simulink subsystem "Dynamics_6DOF_QUAT"  (R2024b)
settings: Solver=VariableStepAuto  StartTime=0.0  StopTime=10.0  RelTol=1e-3
undefined symbols (not defined in the file): Earth, F, fractalcoef, GC, GlobalPosition, Light, MIL, Parameters, WGS84
libraries: aerolibwind2 x3, sharedtransform x2, robotcorelib x2, shared6dof x1, aerolibatmos2 x1, mspfiltlib x1, simulink x1, aerolibasang x1, aerolibtransform2 x1, eeGeneralControl x1, simulink_extras x1, sensorgpslib x1
settings Model: Creator=thesa  LastModifiedBy=jack
settings RTWCC: GPUComputeCapability=3.5

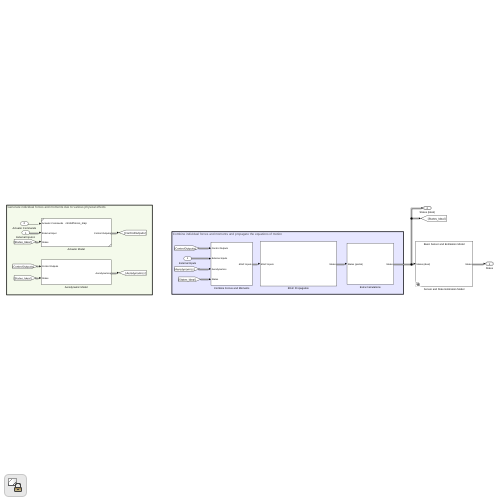
[thumbnail: Simulink's stored preview of the top-level diagram]
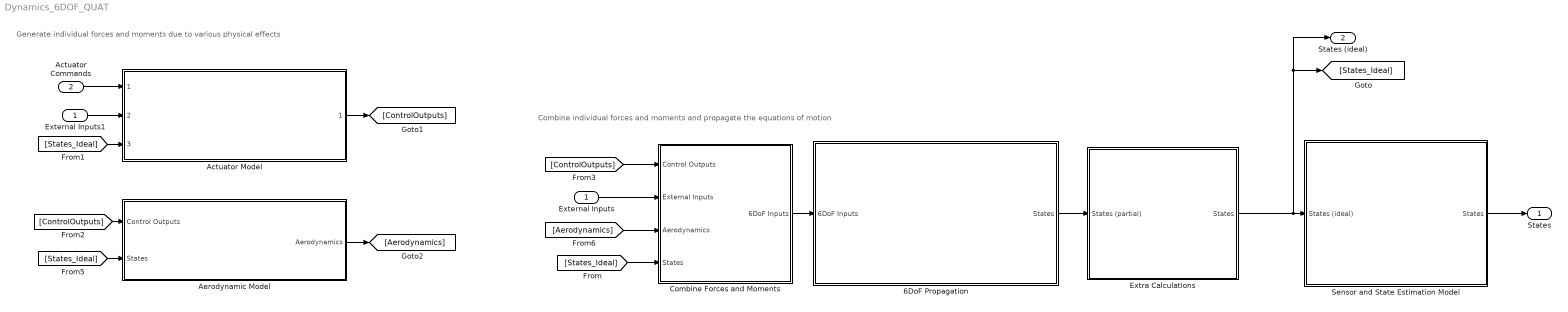
== system Dynamics_6DOF_QUAT ==
  note: Combine individual forces and moments and propagate the equations of motion
  note: Generate individual forces and moments due to various physical effects
  External Inputs : Inport
  Actuator Commands : Inport  Port=2
  6DoF Propagation : Subsystem
  Actuator Model : Subsystem  ReferencedSubsystem=cmds2forces_map
  Aerodynamic Model : Subsystem
  Combine Forces and Moments : Subsystem
  External Inputs1 : InportShadow
  Extra Calculations : Subsystem
  Sensor and State Estimation Model : Subsystem  Variant=on  VariantControlMode=label  VariantControl=Sensor and State Estimation Model  LabelModeActiveChoice=Full Sensor and Estimation Model1
  States : Outport  OutDataTypeStr=Bus: States
  States (ideal) : Outport  Port=2  OutDataTypeStr=Bus: States
  wires:
  6DoF Propagation/1(States) -> Extra Calculations/1(States (partial))
  [ControlOutputs] -> Combine Forces and Moments/1(Control Outputs)
  External Inputs/1 -> Combine Forces and Moments/2(External Inputs)
  [States_Ideal] -> Combine Forces and Moments/4(States)
  [States_Ideal] -> Aerodynamic Model/2(States)
  [ControlOutputs] -> Aerodynamic Model/1(Control Outputs)
  Actuator Model/1 -> [ControlOutputs]
  [States_Ideal] -> Actuator Model/3
  Aerodynamic Model/1(Aerodynamics) -> [Aerodynamics]
  [Aerodynamics] -> Combine Forces and Moments/3(Aerodynamics)
  External Inputs1/1 -> Actuator Model/2
  Actuator Commands/1 -> Actuator Model/1
  Combine Forces and Moments/1(6DoF Inputs) -> 6DoF Propagation/1(6DoF Inputs)
  Sensor and State Estimation Model/1(States) -> States/1
  Extra Calculations/1(States) -> Sensor and State Estimation Model/1(States (ideal)), [States_Ideal], States (ideal)/1

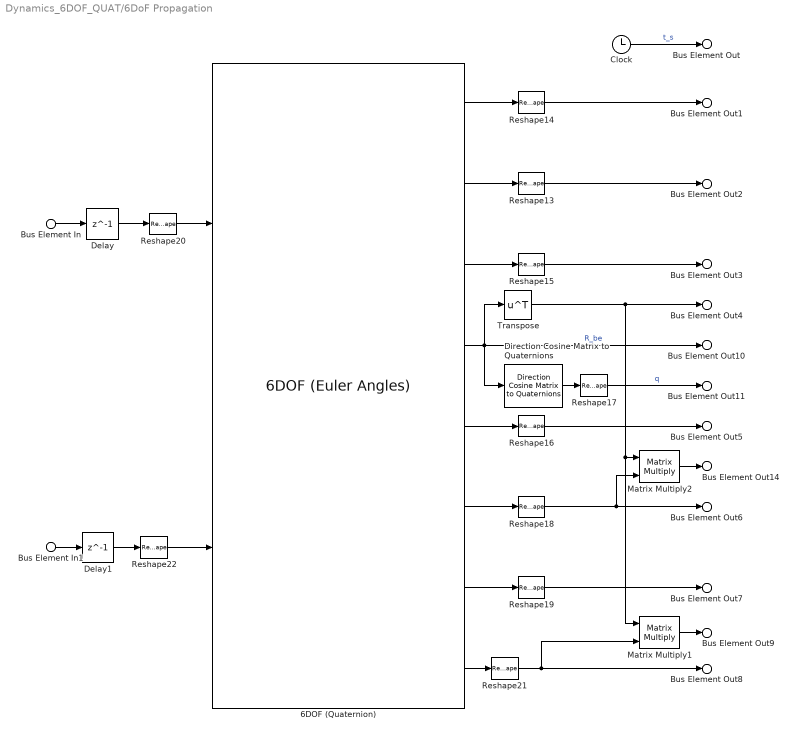
== system Dynamics_6DOF_QUAT/6DoF Propagation ==
  Bus Element In : Inport  PortName=6DoF Inputs  Element=F_body
  Bus Element In1 : Inport  PortName=6DoF Inputs  Element=M_body
  6DOF (Quaternion) : shared6dof/6DOF (Euler Angles)  units=Metric (MKS)  mtype=Fixed  rep=Quaternion  xme_0=p_0  Vm_0=v_0  eul_0=att_0  pm_0=omega_0  mass_0=Parameters.Vehicle.m  mass_e=0.5  mass_f=2.0  inertia=Parameters.Vehicle.I  inertia_e=eye(3)  inertia_f=2*eye(3)  k_quat=1.0  vre_flag=on  abi_flag=off  aMode=0  xme_statename=''  Vm_statename=''  eul_statename=''  quat_statename=''  pm_statename=''  mass_statename=''
  Clock : Clock
  Delay : Delay  DelayLength=1
  Delay1 : Delay  DelayLength=1
  Direction Cosine Matrix to Quaternions : sharedtransform/Direction Cosine Matrix  to Quaternions  aMode=0  action=None  tolerance=eps(2)
  Matrix Multiply1 : Product  Multiplication=Matrix(*)
  Matrix Multiply2 : Product  Multiplication=Matrix(*)
  Reshape{13..16,18..22} (9 alike) : Reshape  OutputDimensionality=Column vector (2-D)
  Reshape17 : Reshape  OutputDimensionality=Row vector (2-D)
  Transpose : Math  Operator=transpose
  Bus Element Out : Outport  PortName=States  Element=t_s
  Bus Element Out2 : Outport  PortName=States  Element=p_e
  Bus Element Out1 : Outport  PortName=States  Element=v_e
  Bus Element Out5 : Outport  PortName=States  Element=v_b
  Bus Element Out9 : Outport  PortName=States  Element=a_e
  Bus Element Out8 : Outport  PortName=States  Element=a_b
  Bus Element Out11 : Outport  PortName=States  Element=q
  Bus Element Out3 : Outport  PortName=States  Element=att
  Bus Element Out6 : Outport  PortName=States  Element=omega_b
  Bus Element Out14 : Outport  PortName=States  Element=omega_e
  Bus Element Out7 : Outport  PortName=States  Element=omega_dot
  Bus Element Out4 : Outport  PortName=States  Element=R_eb
  Bus Element Out10 : Outport  PortName=States  Element=R_be
  wires:
  Matrix Multiply2/1 -> Bus Element Out14/1
  Matrix Multiply1/1 -> Bus Element Out9/1
  Reshape19/1 -> Bus Element Out7/1
  Reshape18/1 -> Matrix Multiply2/2, Bus Element Out6/1
  Reshape16/1 -> Bus Element Out5/1
  Reshape17/1 -> Bus Element Out11/1  "q"
  Transpose/1 -> Matrix Multiply1/1, Matrix Multiply2/1, Bus Element Out4/1
  Reshape15/1 -> Bus Element Out3/1
  Reshape13/1 -> Bus Element Out2/1
  Reshape14/1 -> Bus Element Out1/1
  Clock/1 -> Bus Element Out/1  "t_s"
  Delay1/1 -> Reshape22/1
  Direction Cosine Matrix to Quaternions/1 -> Reshape17/1
  Reshape22/1 -> 6DOF (Quaternion)/2
  6DOF (Quaternion)/2 -> Reshape13/1
  6DOF (Quaternion)/8 -> Reshape21/1
  6DOF (Quaternion)/1 -> Reshape14/1
  Bus Element In1/1 -> Delay1/1
  6DOF (Quaternion)/7 -> Reshape19/1
  Reshape21/1 -> Matrix Multiply1/2, Bus Element Out8/1
  6DOF (Quaternion)/4 -> Direction Cosine Matrix to Quaternions/1, Bus Element Out10/1, Transpose/1  "R_be"
  Bus Element In/1 -> Delay/1
  6DOF (Quaternion)/5 -> Reshape16/1
  Reshape20/1 -> 6DOF (Quaternion)/1
  6DOF (Quaternion)/6 -> Reshape18/1
  6DOF (Quaternion)/3 -> Reshape15/1
  Delay/1 -> Reshape20/1

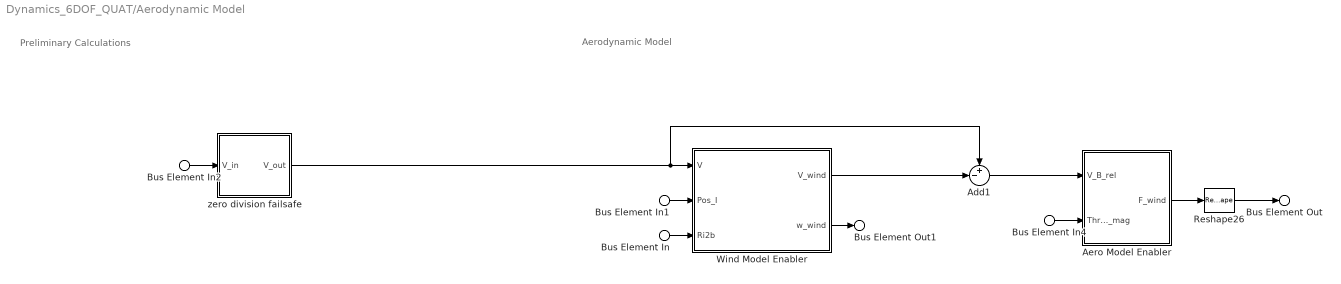
== system Dynamics_6DOF_QUAT/Aerodynamic Model ==
  note: Aerodynamic Model
  note: Preliminary Calculations
  Bus Element In4 : Inport  PortName=Control Outputs  Element=T
  Bus Element In : Inport  Port=2  PortName=States  Element=R_be
  Bus Element In1 : Inport  Port=2  PortName=States  Element=p_e
  Bus Element In2 : Inport  Port=2  PortName=States  Element=v_b
  Add1 : Sum  Inputs=+-|
  Aero Model Enabler : Subsystem
  Reshape26 : Reshape  OutputDimensionality=Column vector (2-D)
  Wind Model Enabler : Subsystem
  zero division failsafe : Subsystem
  Bus Element Out : Outport  PortName=Aerodynamics  Element=F_body
  Bus Element Out1 : Outport  PortName=Aerodynamics  Element=w
  wires:
  Add1/1 -> Aero Model Enabler/1(V_B_rel)
  Bus Element In/1 -> Wind Model Enabler/3(Ri2b)
  Bus Element In1/1 -> Wind Model Enabler/2(Pos_I)
  Bus Element In4/1 -> Aero Model Enabler/2(Thrust_mag)
  Wind Model Enabler/1(V_wind) -> Add1/2
  zero division failsafe/1(V_out) -> Add1/1, Wind Model Enabler/1(V)
  Bus Element In2/1 -> zero division failsafe/1(V_in)
  Wind Model Enabler/2(w_wind) -> Bus Element Out1/1
  Reshape26/1 -> Bus Element Out/1
  Aero Model Enabler/1(F_wind) -> Reshape26/1

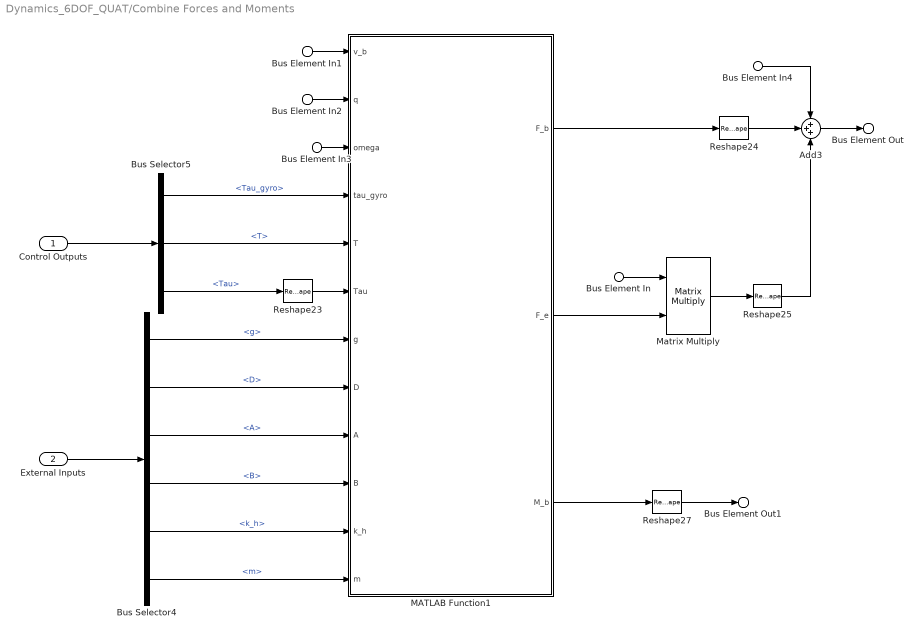
== system Dynamics_6DOF_QUAT/Combine Forces and Moments ==
  Control Outputs : Inport
  External Inputs : Inport  Port=2
  Bus Element In3 : Inport  Port=3  PortName=Aerodynamics  Element=w
  Bus Element In4 : Inport  Port=3  PortName=Aerodynamics  Element=F_body
  Bus Element In : Inport  Port=4  PortName=States  Element=R_be
  Bus Element In1 : Inport  Port=4  PortName=States  Element=v_b
  Bus Element In2 : Inport  Port=4  PortName=States  Element=q
  Add3 : Sum  Inputs=+++
  Bus Selector4 : BusSelector  OutputSignals=Vehicle Parameters.g,Vehicle Parameters.D,Vehicle Parameters.A,Vehicle Parameters.B,Vehicle Parameters.k_h,Vehicle Parameters.m
  Bus Selector5 : BusSelector  OutputSignals=Tau_gyro,T,Tau
  MATLAB Function1 : MATLAB Function  TreatAsAtomicUnit=on
  Matrix Multiply : Product  Multiplication=Matrix(*)
  Reshape{23..25,27} (4 alike) : Reshape  OutputDimensionality=Column vector (2-D)
  Bus Element Out : Outport  PortName=6DoF Inputs  Element=F_body
  Bus Element Out1 : Outport  PortName=6DoF Inputs  Element=M_body
  wires:
  Add3/1 -> Bus Element Out/1
  Bus Element In4/1 -> Add3/1
  Bus Element In/1 -> Matrix Multiply/1
  Reshape25/1 -> Add3/3
  Reshape24/1 -> Add3/2
  Bus Selector5/3 -> Reshape23/1  "<Tau>"
  Bus Element In3/1 -> MATLAB Function1/3(omega)
  Bus Selector4/5 -> MATLAB Function1/11(k_h)  "<k_h>"
  External Inputs/1 -> Bus Selector4/1
  Bus Element In1/1 -> MATLAB Function1/1(v_b)
  Bus Selector4/3 -> MATLAB Function1/9(A)  "<A>"
  Bus Selector4/2 -> MATLAB Function1/8(D)  "<D>"
  Bus Selector5/1 -> MATLAB Function1/4(tau_gyro)  "<Tau_gyro>"
  Bus Element In2/1 -> MATLAB Function1/2(q)
  MATLAB Function1/1(F_b) -> Reshape24/1
  Bus Selector4/6 -> MATLAB Function1/12(m)  "<m>"
  Reshape27/1 -> Bus Element Out1/1
  Matrix Multiply/1 -> Reshape25/1
  MATLAB Function1/2(F_e) -> Matrix Multiply/2
  Reshape23/1 -> MATLAB Function1/6(Tau)
  Bus Selector5/2 -> MATLAB Function1/5(T)  "<T>"
  Bus Selector4/1 -> MATLAB Function1/7(g)  "<g>"
  MATLAB Function1/3(M_b) -> Reshape27/1
  Control Outputs/1 -> Bus Selector5/1
  Bus Selector4/4 -> MATLAB Function1/10(B)  "<B>"

== system Dynamics_6DOF_QUAT/Extra Calculations ==
  States (partial) : Inport
  AirData : Subsystem  ReferencedSubsystem=AirData
  Bus Assignment : BusAssignment  AssignedSignals=GlobalPosition,GC
  Bus Assignment1 : BusAssignment  AssignedSignals=AirData
  GlobalPosition : Subsystem  ReferencedSubsystem=GlobalPosition
  Ground Contact Model : Subsystem  ReferencedSubsystem=Ground_Contact_Model
  States : Outport
  wires:
  Bus Assignment1/1 -> States/1
  AirData/1 -> Bus Assignment1/2
  Bus Assignment/1 -> Bus Assignment1/1, AirData/1
  Ground Contact Model/1 -> Bus Assignment/3
  GlobalPosition/1 -> Bus Assignment/2
  States (partial)/1 -> Bus Assignment/1, GlobalPosition/1, Ground Contact Model/1

== system Dynamics_6DOF_QUAT/Sensor and State Estimation Model ==
  States (ideal) : Inport
  Basic Sensor and Estimation Model : Subsystem  VariantControl=Full Sensor and Estimation Model1
  Ideal : Subsystem  VariantControl=Sensor and State Estimation Model
  States : Outport

== system Dynamics_6DOF_QUAT/Aerodynamic Model/Aero Model Enabler ==
  V_B_rel : Inport
  Thrust_mag : Inport  Port=2
  Constant : Constant  Value=Parameters.Simulink.EN_AERO_MODEL
  If : If  IfExpression=u1
  If Action Subsystem1 : Subsystem  TreatAsAtomicUnit=on
  Merge : Merge
  Reshape3 : Reshape
  To Workspace1 : ToWorkspace  VariableName=wind_F  SampleTime=-1
  zero force : Subsystem  TreatAsAtomicUnit=on
  F_wind : Outport
  wires:
  Merge/1 -> F_wind/1, Reshape3/1
  If Action Subsystem1/1(F_wind) -> Merge/2
  zero force/1(Out1) -> Merge/1
  Constant/1 -> If/1
  If/1 -> If Action Subsystem1/Action
  Reshape3/1 -> To Workspace1/1
  V_B_rel/1 -> If Action Subsystem1/1(V_B_rel)
  If/2 -> zero force/Action
  Thrust_mag/1 -> If Action Subsystem1/2(Thrust_mag)

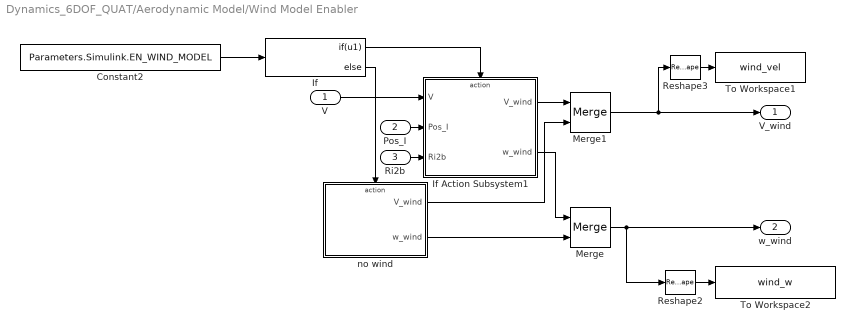
== system Dynamics_6DOF_QUAT/Aerodynamic Model/Wind Model Enabler ==
  V : Inport
  Pos_I : Inport  Port=2
  Ri2b : Inport  Port=3
  Constant2 : Constant  Value=Parameters.Simulink.EN_WIND_MODEL
  If : If  IfExpression=u1
  If Action Subsystem1 : Subsystem  TreatAsAtomicUnit=on
  Merge : Merge
  Merge1 : Merge
  Reshape2 : Reshape
  Reshape3 : Reshape
  To Workspace1 : ToWorkspace  VariableName=wind_vel  SampleTime=-1
  To Workspace2 : ToWorkspace  VariableName=wind_w  SampleTime=-1
  no wind : Subsystem  TreatAsAtomicUnit=on
  V_wind : Outport
  w_wind : Outport  Port=2
  wires:
  If Action Subsystem1/1(V_wind) -> Merge1/1
  If/1 -> If Action Subsystem1/Action
  Constant2/1 -> If/1
  Merge/1 -> w_wind/1, Reshape2/1
  V/1 -> If Action Subsystem1/1(V)
  If Action Subsystem1/2(w_wind) -> Merge/1
  If/2 -> no wind/Action
  no wind/1(V_wind) -> Merge1/2
  no wind/2(w_wind) -> Merge/2
  Merge1/1 -> Reshape3/1, V_wind/1
  Reshape2/1 -> To Workspace2/1
  Reshape3/1 -> To Workspace1/1
  Pos_I/1 -> If Action Subsystem1/2(Pos_I)
  Ri2b/1 -> If Action Subsystem1/3(Ri2b)

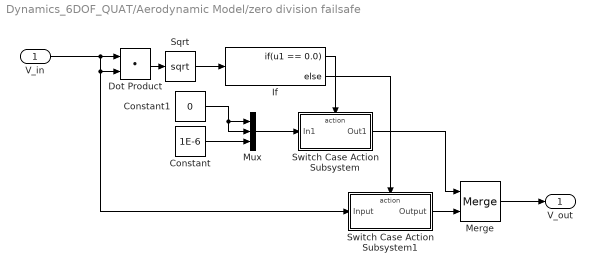
== system Dynamics_6DOF_QUAT/Aerodynamic Model/zero division failsafe ==
  V_in : Inport
  Constant : Constant  Value=1E-6
  Constant1 : Constant  Value=0
  Dot Product : DotProduct  OutDataTypeStr=Inherit: Inherit via internal rule
  If : If  IfExpression=u1 == 0.0
  Merge : Merge
  Mux : Mux  Inputs=3
  Sqrt : Sqrt
  Switch Case Action Subsystem : Subsystem  TreatAsAtomicUnit=on
  Switch Case Action Subsystem1 : Subsystem  TreatAsAtomicUnit=on
  V_out : Outport
  wires:
  Sqrt/1 -> If/1
  Constant1/1 -> Mux/1, Mux/2
  If/2 -> Switch Case Action Subsystem1/Action
  Mux/1 -> Switch Case Action Subsystem/1(In1)
  Dot Product/1 -> Sqrt/1
  Switch Case Action Subsystem/1(Out1) -> Merge/1
  V_in/1 -> Switch Case Action Subsystem1/1(Input), Dot Product/2, Dot Product/1
  Constant/1 -> Mux/3
  Switch Case Action Subsystem1/1(Output) -> Merge/2
  If/1 -> Switch Case Action Subsystem/Action
  Merge/1 -> V_out/1

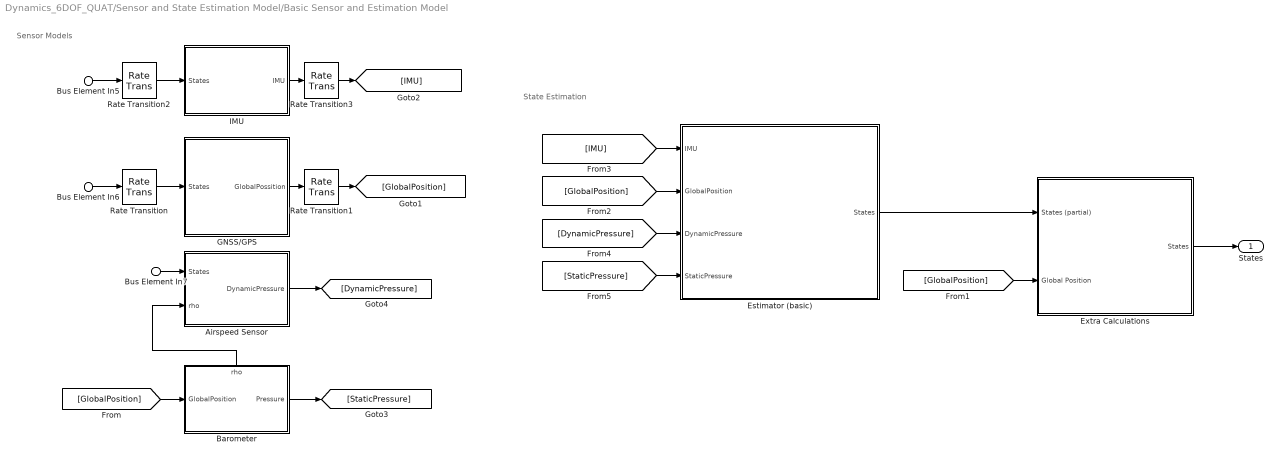
== system Dynamics_6DOF_QUAT/Sensor and State Estimation Model/Basic Sensor and Estimation Model ==
  note: Sensor Models
  note: State Estimation
  Bus Element In5 : Inport  PortName=States (ideal)
  Bus Element In6 : Inport  PortName=States (ideal)
  Bus Element In7 : Inport  PortName=States (ideal)
  " Barometer" : Subsystem
      settings: PortSchema="{\"entries\":[{\"content\":{\"sides\":[{\"content\":{\"connectorIds\":[\"In1\"]},\"type\":\"ConnectorPlacement.EquallySpacedRectSide\",\"uuid\":\"98aeca60-ddc5-44bc-b6e2-5cf50dbbc9ef\"},{\"content\":{\"connectorIds\":[\"Out1\"],\"side\":\"RIGHT\"},\"type\":\"ConnectorPlacement.EquallySpacedRectSide\",\"uuid\":\"ee7488f2-91e3-47d4-9081-a46159bb1103\"},{\"content\":{\"connectorIds\":[\"Out2\"],\"side\":\"TOP\"},\"type\":\"ConnectorPlacement.EquallySpacedRectSide\",\"uuid\":\"ef0f5ebc-65ee-4ea2-b0e3-56f3f8c3efb6\"}]},\"type\":\"ConnectorPlacement.EquallySpacedConnector\",\"uuid\":\"587852e8-f26f-43d3-aef8-bd8c21ac36ee\"}],\"packageUris\":[\"http://schema.mathworks.com/mf0/Connector/R2020b\"],\"version\":\"1.0\"}"
  Airspeed Sensor : Subsystem
  Estimator (basic) : Subsystem
  Extra Calculations : Subsystem
  GNSS/GPS : Subsystem
  IMU : Subsystem
  Rate Transition{,1..3} (4 alike) : RateTransition  OutPortSampleTime=Parameters.Simulink.time_step_s
  States : Outport
  wires:
  Extra Calculations/1(States) -> States/1
  Bus Element In7/1 -> Airspeed Sensor/1(States)
  Bus Element In6/1 -> Rate Transition/1
  Rate Transition2/1 -> IMU/1(States)
  Bus Element In5/1 -> Rate Transition2/1
  Rate Transition1/1 -> [GlobalPosition]
  Rate Transition/1 -> GNSS/GPS/1(States)
  Rate Transition3/1 -> [IMU]
  GNSS/GPS/1(GlobalPossition) -> Rate Transition1/1
  [StaticPressure] -> Estimator (basic)/4(StaticPressure)
  [DynamicPressure] -> Estimator (basic)/3(DynamicPressure)
  [GlobalPosition] -> Extra Calculations/2(Global Position)
  Estimator (basic)/1(States) -> Extra Calculations/1(States (partial))
  [GlobalPosition] -> Estimator (basic)/2(GlobalPosition)
  [IMU] -> Estimator (basic)/1(IMU)
  IMU/1(IMU) -> Rate Transition3/1
  [GlobalPosition] -> " Barometer"/1(GlobalPosition)
  " Barometer"/2(rho) -> Airspeed Sensor/2(rho)
  Airspeed Sensor/1(DynamicPressure) -> [DynamicPressure]
  " Barometer"/1(Pressure) -> [StaticPressure]

== system Dynamics_6DOF_QUAT/Sensor and State Estimation Model/Ideal ==
  States (ideal) : Inport
  States : Outport
  wires:
  States (ideal)/1 -> States/1

== system Dynamics_6DOF_QUAT/Aerodynamic Model/Aero Model Enabler/If Action Subsystem1 ==
  V_B_rel : Inport
  Thrust_mag : Inport  Port=2
  Action Port : ActionPort
  Aerodynamic Model : Subsystem
  F_wind : Outport
  wires:
  V_B_rel/1 -> Aerodynamic Model/2(V_B_rel)
  Aerodynamic Model/1(F_wind) -> F_wind/1
  Thrust_mag/1 -> Aerodynamic Model/1(Thrust_mag)

== system Dynamics_6DOF_QUAT/Aerodynamic Model/Aero Model Enabler/zero force ==
  Action Port : ActionPort
  Constant : Constant  Value=zeros(3,1)
  Out1 : Outport
  wires:
  Constant/1 -> Out1/1

== system Dynamics_6DOF_QUAT/Aerodynamic Model/Wind Model Enabler/If Action Subsystem1 ==
  V : Inport
  Pos_I : Inport  Port=2
  Ri2b : Inport  Port=3
  Action Port : ActionPort
  Wind Model : Subsystem
  V_wind : Outport
  w_wind : Outport  Port=2
  wires:
  Wind Model/1(V_wind) -> V_wind/1
  Wind Model/2(Omega wind) -> w_wind/1
  Pos_I/1 -> Wind Model/1(Position)
  Ri2b/1 -> Wind Model/3(Ri2b)
  V/1 -> Wind Model/2(Velocity)

== system Dynamics_6DOF_QUAT/Aerodynamic Model/Wind Model Enabler/no wind ==
  Action Port : ActionPort
  Constant : Constant  Value=zeros(3,1)
  V_wind : Outport
  w_wind : Outport  Port=2
  wires:
  Constant/1 -> w_wind/1, V_wind/1

== system Dynamics_6DOF_QUAT/Aerodynamic Model/zero division failsafe/Switch Case Action Subsystem ==
  In1 : Inport
  Action Port : ActionPort
  Out1 : Outport
  wires:
  In1/1 -> Out1/1

== system Dynamics_6DOF_QUAT/Aerodynamic Model/zero division failsafe/Switch Case Action Subsystem1 ==
  Input : Inport
  Action Port : ActionPort
  Output : Outport
  wires:
  Input/1 -> Output/1

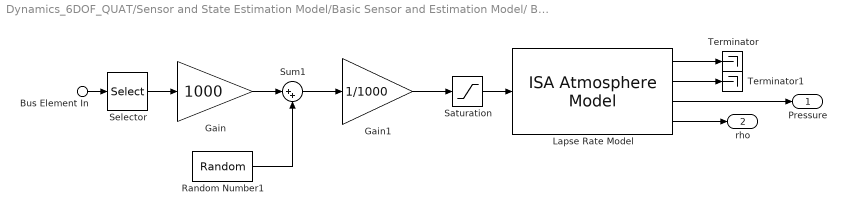
== system Dynamics_6DOF_QUAT/Sensor and State Estimation Model/Basic Sensor and Estimation Model/ Barometer ==
  Bus Element In : Inport  PortName=GlobalPosition  Element=LLA
  Gain : Gain  Gain=1000
  Gain1 : Gain  Gain=1/1000
  Lapse Rate Model : aerolibatmos2/ISA Atmosphere Model  useExtended=off  action=Warning  custom=on  viscosityOut=off  g=9.80665  gamma=1.4  R=287.0531  L=0.0065  h_trop=11000  h_strat=20000  rho0=1.225  P0=101325  T0=288.15  h0=0  S=110.4  Tref=273.15  muref=1.716e-5
  Random Number1 : RandomNumber  Variance=10  Seed=10  SampleTime=Parameters.Simulink.time_step_s
  Saturation : Saturate  UpperLimit=20000  LowerLimit=0
  Selector : Selector  InputPortWidth=3  IndexOptions=Index vector (dialog)  Indices=3  OutputSizes=1
  Sum1 : Sum  Inputs=|++
  Terminator : Terminator
  Terminator1 : Terminator
  Pressure : Outport
  rho : Outport  Port=2
  wires:
  Saturation/1 -> Lapse Rate Model/1
  Gain/1 -> Sum1/1
  Random Number1/1 -> Sum1/2
  Gain1/1 -> Saturation/1
  Bus Element In/1 -> Selector/1
  Selector/1 -> Gain/1
  Sum1/1 -> Gain1/1
  Lapse Rate Model/3 -> Pressure/1
  Lapse Rate Model/1 -> Terminator/1
  Lapse Rate Model/4 -> rho/1
  Lapse Rate Model/2 -> Terminator1/1

== system Dynamics_6DOF_QUAT/Sensor and State Estimation Model/Basic Sensor and Estimation Model/Airspeed Sensor ==
  In Bus Element : Inport  PortName=States  Element=AirData.Airspeed
  rho : Inport  Port=2
  Constant : Constant  Value=0.5
  Constant1 : Constant  Value=0
  Max : MinMax  Function=max  Inputs=2
  Product : Product  Inputs=3
  Random Number1 : RandomNumber  Variance=0.1  Seed=545  SampleTime=Parameters.Simulink.time_step_s
  Square : Math  Operator=square
  Sum : Sum  Inputs=|++
  DynamicPressure : Outport
  wires:
  Constant1/1 -> Max/2
  Sum/1 -> Max/1
  Max/1 -> DynamicPressure/1
  Random Number1/1 -> Sum/2  "Pressure_noise"
  Product/1 -> Sum/1
  In Bus Element/1 -> Square/1
  Square/1 -> Product/1
  rho/1 -> Product/2
  Constant/1 -> Product/3

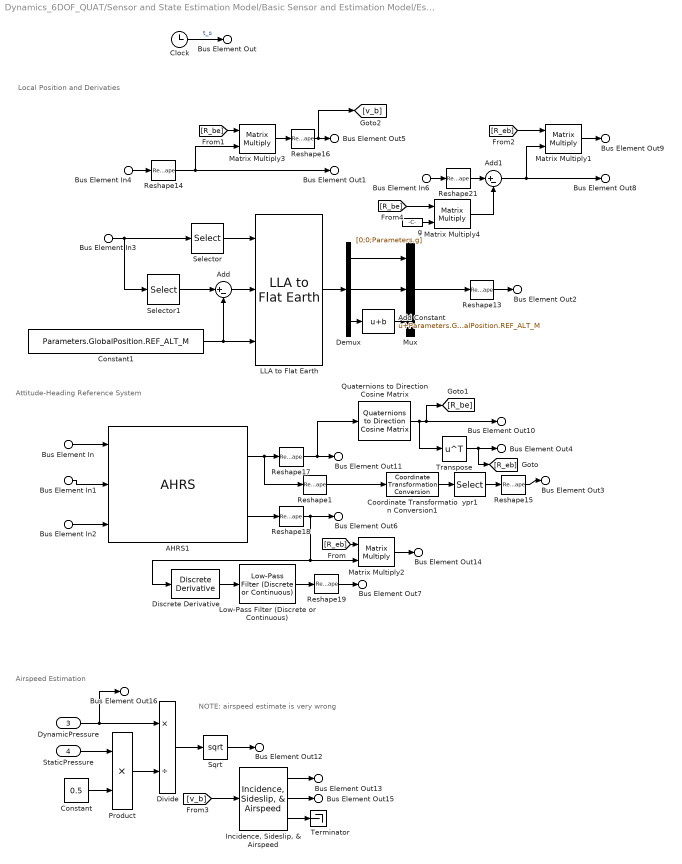
== system Dynamics_6DOF_QUAT/Sensor and State Estimation Model/Basic Sensor and Estimation Model/Estimator (basic) ==
  note: Local Position and Derivaties
  note: Attitude-Heading Reference System
  note: Airspeed Estimation
  note: NOTE: airspeed estimate is very wrong
  Bus Element In : Inport  PortName=IMU  Element=Accel
  Bus Element In6 : Inport  PortName=IMU  Element=Accel
  Bus Element In1 : Inport  PortName=IMU  Element=Gyro
  Bus Element In2 : Inport  PortName=IMU  Element=Mag
  Bus Element In3 : Inport  Port=2  PortName=GlobalPosition  Element=LLA
  Bus Element In4 : Inport  Port=2  PortName=GlobalPosition  Element=V_e
  DynamicPressure : Inport  Port=3
  StaticPressure : Inport  Port=4
  AHRS1 : mspfiltlib/AHRS  DispRefFrame=NED  DecimationFactor=1  InitialProcessNoise=ahrsfilter.defaultProcessNoise  OrientationFormat=quaternion  SimulateUsing=Code generation  AccelerometerNoise=0.0001924722  GyroscopeNoise=9.1385e-5  MagnetometerNoise=0.1  GyroscopeDriftNoise=3.0462e-13  LinearAccelerationNoise=0.0096236100000000012  MagneticDisturbanceNoise=0.5  LinearAccelerationDecayFactor=0.998  MagneticDisturbanceDecayFactor=0.5  ExpectedMagneticFieldStrength=40
  Add : Sum  Inputs=|+-
  Add Constant : Bias  Bias=Parameters.GlobalPosition.REF_ALT_M  SaturateOnIntegerOverflow=off
  Add1 : Sum  Inputs=|+-
  Clock : Clock
  Constant : Constant  Value=0.5
  Constant1 : Constant  Value=Parameters.GlobalPosition.REF_ALT_M
  Coordinate Transformation Conversion1 : robotcorelib/Coordinate Transformation Conversion  InputRepresentation=Quaternion  InputEulerSequence=ZYX  ShowTrVecInputPort=on  OutputRepresentation=Euler Angles  OutputEulerSequence=ZYX  ShowTrVecOutputPort=on  SimulateUsing=Interpreted execution
  Demux : Demux  Outputs=3
  Discrete Derivative : simulink/Discrete/Discrete Derivative  gainval=1.0  ICPrevScaledInput=0.0  OutMin=[]  OutMax=[]  OutDataType=fixdt(1, 16)  OutScaling=2^-10  DoSatur=off
  Divide : Product  Inputs=*/
  "Incidence, Sideslip, & Airspeed" : aerolibasang/Incidence, Sideslip, & Airspeed
  LLA to Flat Earth : aerolibtransform2/LLA to Flat Earth  units=Metric (MKS)  ptype=Earth (WGS84)  F=1/298.257223563  R=6378137  refPosPort=off  LL0=[Parameters.GlobalPosition.REF_LAT_DEG, Parameters.GlobalPosition.REF_LONG_DEG]  psi=0
  Low-Pass Filter (Discrete or Continuous) : eeGeneralControl/Low-Pass Filter (Discrete or Continuous)  K=1  T=1/10  B=inf  A=-inf  init_option=Inherited from block input  x0=0  Ts=-1
  Matrix Multiply{1..4} (4 alike) : Product  Multiplication=Matrix(*)
  Mux : Mux  Inputs=3
  Product : Product
  Quaternions to Direction Cosine Matrix : sharedtransform/Quaternions to  Direction Cosine Matrix  aMode=aMode
  Reshape{1,13..16,18..19,21} (8 alike) : Reshape  OutputDimensionality=Column vector (2-D)
  Reshape17 : Reshape  OutputDimensionality=Row vector (2-D)
  Selector : Selector  InputPortWidth=3  IndexOptions=Index vector (dialog)  Indices=[1,2]  OutputSizes=1
  Selector1 : Selector  InputPortWidth=3  IndexOptions=Index vector (dialog)  Indices=3  OutputSizes=1
  Sqrt : Sqrt
  Terminator : Terminator
  Transpose : Math  Operator=transpose
  g : Constant  Value=[0;0;Parameters.g]
  ypr1 : Selector  InputPortWidth=3  IndexOptions=Index vector (dialog)  Indices=[3 2 1]  OutputSizes=1
  Bus Element Out : Outport  PortName=States  Element=t_s
  Bus Element Out2 : Outport  PortName=States  Element=p_e
  Bus Element Out1 : Outport  PortName=States  Element=v_e
  Bus Element Out5 : Outport  PortName=States  Element=v_b
  Bus Element Out9 : Outport  PortName=States  Element=a_e
  Bus Element Out8 : Outport  PortName=States  Element=a_b
  Bus Element Out11 : Outport  PortName=States  Element=q
  Bus Element Out3 : Outport  PortName=States  Element=att
  Bus Element Out6 : Outport  PortName=States  Element=omega_b
  Bus Element Out14 : Outport  PortName=States  Element=omega_e
  Bus Element Out7 : Outport  PortName=States  Element=omega_dot
  Bus Element Out4 : Outport  PortName=States  Element=R_eb
  Bus Element Out10 : Outport  PortName=States  Element=R_be
  Bus Element Out13 : Outport  PortName=States  Element=AirData.AoA
  Bus Element Out15 : Outport  PortName=States  Element=AirData.Beta
  Bus Element Out12 : Outport  PortName=States  Element=AirData.Airspeed
  Bus Element Out16 : Outport  PortName=States  Element=AirData.q
  wires:
  Matrix Multiply4/1 -> Add1/2
  Reshape21/1 -> Add1/1
  [R_be] -> Matrix Multiply4/1
  g/1 -> Matrix Multiply4/2
  Mux/1 -> Reshape13/1
  Add Constant/1 -> Mux/3
  Demux/3 -> Add Constant/1
  Demux/1 -> Mux/1
  Demux/2 -> Mux/2
  Add/1 -> LLA to Flat Earth/2
  Reshape1/1 -> Coordinate Transformation Conversion1/1
  Discrete Derivative/1 -> Low-Pass Filter (Discrete or Continuous)/1
  Reshape18/1 -> Bus Element Out6/1, Matrix Multiply2/2, Discrete Derivative/1
  [v_b] -> "Incidence, Sideslip, & Airspeed"/1
  "Incidence, Sideslip, & Airspeed"/3 -> Terminator/1
  "Incidence, Sideslip, & Airspeed"/2 -> Bus Element Out15/1
  "Incidence, Sideslip, & Airspeed"/1 -> Bus Element Out13/1
  Constant/1 -> Product/2
  StaticPressure/1 -> Product/1
  Product/1 -> Divide/2
  DynamicPressure/1 -> Divide/1, Bus Element Out16/1
  Divide/1 -> Sqrt/1
  Sqrt/1 -> Bus Element Out12/1
  [R_eb] -> Matrix Multiply1/1
  [R_be] -> Matrix Multiply3/1
  Reshape14/1 -> Bus Element Out1/1, Matrix Multiply3/2
  [R_eb] -> Matrix Multiply2/1
  Quaternions to Direction Cosine Matrix/1 -> Transpose/1, [R_be], Bus Element Out10/1
  Reshape15/1 -> Bus Element Out3/1
  ypr1/1 -> Reshape15/1
  Coordinate Transformation Conversion1/1 -> ypr1/1
  Selector1/1 -> Add/1
  Bus Element In3/1 -> Selector1/1, Selector/1
  Selector/1 -> LLA to Flat Earth/1
  Constant1/1 -> LLA to Flat Earth/3, Add/2
  Bus Element In2/1 -> AHRS1/3
  Bus Element In1/1 -> AHRS1/2
  Bus Element In/1 -> AHRS1/1
  Reshape13/1 -> Bus Element Out2/1
  Bus Element In6/1 -> Reshape21/1
  Matrix Multiply1/1 -> Bus Element Out9/1
  LLA to Flat Earth/1 -> Demux/1
  Low-Pass Filter (Discrete or Continuous)/1 -> Reshape19/1
  Reshape17/1 -> Bus Element Out11/1, Quaternions to Direction Cosine Matrix/1
  AHRS1/2 -> Reshape18/1
  AHRS1/1 -> Reshape1/1, Reshape17/1
  Bus Element In4/1 -> Reshape14/1
  Transpose/1 -> Bus Element Out4/1, [R_eb]
  Matrix Multiply3/1 -> Reshape16/1
  Reshape19/1 -> Bus Element Out7/1
  Add1/1 -> Matrix Multiply1/2, Bus Element Out8/1
  Clock/1 -> Bus Element Out/1  "t_s"
  Reshape16/1 -> Bus Element Out5/1, [v_b]
  Matrix Multiply2/1 -> Bus Element Out14/1

== system Dynamics_6DOF_QUAT/Sensor and State Estimation Model/Basic Sensor and Estimation Model/Extra Calculations ==
  States (partial) : Inport
  Global Position : Inport  Port=2
  Bus Assignment : BusAssignment  AssignedSignals=GC,GlobalPosition
  Ground Contact Model : Subsystem  ReferencedSubsystem=Ground_Contact_Model
  States : Outport
  wires:
  Ground Contact Model/1 -> Bus Assignment/2
  Bus Assignment/1 -> States/1
  Global Position/1 -> Bus Assignment/3
  States (partial)/1 -> Bus Assignment/1, Ground Contact Model/1

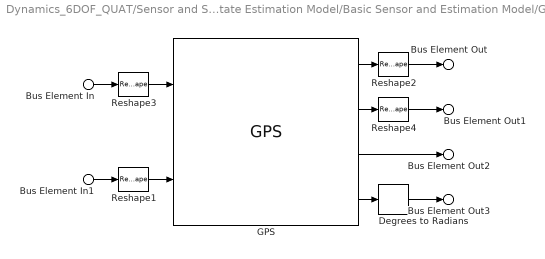
== system Dynamics_6DOF_QUAT/Sensor and State Estimation Model/Basic Sensor and Estimation Model/GNSS//GPS ==
  Bus Element In : Inport  PortName=States  Element=p_e
  Bus Element In1 : Inport  PortName=States  Element=v_e
  Degrees to Radians : simulink_extras/Transformations/Degrees to Radians
  GPS : sensorgpslib/GPS  DispRefFrame=NED  PositionInputFormat=Local  ReferenceLocation=[Parameters.GlobalPosition.REF_LAT_DEG, Parameters.GlobalPosition.REF_LONG_DEG, Parameters.GlobalPosition.REF_ALT_M]  HorizontalPositionAccuracy=0.01  VerticalPositionAccuracy=0.01  VelocityAccuracy=0.01  DecayFactor=0  SeedDouble=67  SimulateUsing=Code generation
      settings: LibrarySourceBlock=uavsimlib/GPS
  Reshape1 : Reshape  OutputDimensionality=Row vector (2-D)
  Reshape2 : Reshape  OutputDimensionality=Column vector (2-D)
  Reshape3 : Reshape  OutputDimensionality=Row vector (2-D)
  Reshape4 : Reshape  OutputDimensionality=Column vector (2-D)
  Bus Element Out : Outport  PortName=GlobalPossition  Element=LLA
  Bus Element Out1 : Outport  PortName=GlobalPossition  Element=V_e
  Bus Element Out2 : Outport  PortName=GlobalPossition  Element=GroundSpeed
  Bus Element Out3 : Outport  PortName=GlobalPossition  Element=Course
  wires:
  Reshape2/1 -> Bus Element Out/1
  Bus Element In/1 -> Reshape3/1
  Bus Element In1/1 -> Reshape1/1
  GPS/4 -> Degrees to Radians/1
  GPS/3 -> Bus Element Out2/1
  GPS/2 -> Reshape4/1
  GPS/1 -> Reshape2/1
  Reshape3/1 -> GPS/1
  Reshape1/1 -> GPS/2
  Degrees to Radians/1 -> Bus Element Out3/1
  Reshape4/1 -> Bus Element Out1/1

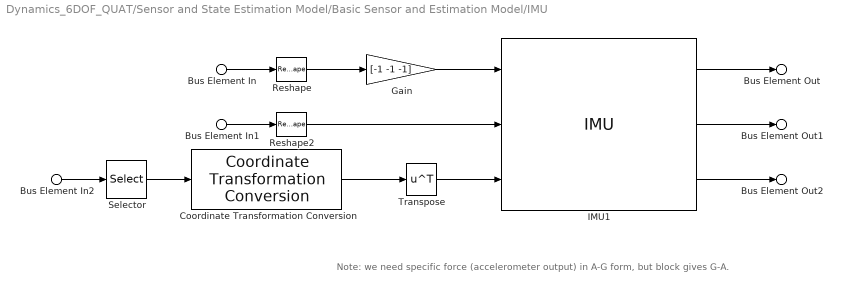
== system Dynamics_6DOF_QUAT/Sensor and State Estimation Model/Basic Sensor and Estimation Model/IMU ==
  note: Note:
      | we need specific force (accelerometer output) in A-G form, but block gives G-A.
  Bus Element In : Inport  PortName=States  Element=a_e
  Bus Element In2 : Inport  PortName=States  Element=att
  Bus Element In1 : Inport  PortName=States  Element=omega_e
  Coordinate Transformation Conversion : robotcorelib/Coordinate Transformation Conversion  InputRepresentation=Euler Angles  InputEulerSequence=ZYX  ShowTrVecInputPort=on  OutputRepresentation=Rotation Matrix  OutputEulerSequence=ZYX  ShowTrVecOutputPort=on  SimulateUsing=Code generation
  Gain : Gain  Gain=[-1 -1 -1]
  IMU1 : mspsensorlib/IMU  DispRefFrame=NED  TemperaturePort=off  Temperature=25  MagneticFieldPort=off  MagneticFieldNED=[27.5550,-2.4169,-16.0849]  MagneticFieldENU=[ -2.4169, 27.5550, 16.0849 ]  SeedDouble=87254  SimulateUsing=Code generation  AccelParamsMeasurementRange=Inf  AccelParamsResolution=0  AccelParamsConstantBias=[ 0, 0, 0 ]  AccelParamsAxesMisalignment=[ 0, 0, 0 ]  AccelParamsNoiseDensity=0.0003  AccelParamsBiasInstability=[ 0, 0, 0 ]  AccelParamsBiasInstabilityNumerator=fractalcoef().Numerator  AccelParamsBiasInstabilityDenominator=fractalcoef().Denominator  AccelParamsRandomWalk=[ 0, 0, 0 ]  AccelParamsNoiseType=double-sided  AccelParamsTemperatureBias=[ 0, 0, 0 ]  AccelParamsTemperatureScaleFactor=[ 0, 0, 0 ]  GyroParamsMeasurementRange=Inf  GyroParamsResolution=0  GyroParamsConstantBias=[ 0, 0, 0 ]  GyroParamsAxesMisalignment=[ 0, 0, 0 ]  GyroParamsAccelerationBias=0.0001  GyroParamsNoiseDensity=0.0002  GyroParamsBiasInstability=[ 0, 0, 0 ]  GyroParamsBiasInstabilityNumerator=fractalcoef().Numerator  GyroParamsBiasInstabilityDenominator=fractalcoef().Denominator  GyroParamsRandomWalk=[ 0, 0, 0 ]  GyroParamsNoiseType=double-sided  GyroParamsTemperatureBias=[ 0, 0, 0 ]  GyroParamsTemperatureScaleFactor=[ 0, 0, 0 ]  MagParamsMeasurementRange=Inf  MagParamsResolution=0  MagParamsConstantBias=[ 0, 0, 0 ]  MagParamsAxesMisalignment=[ 0, 0, 0 ]  MagParamsNoiseDensity=0.0005  MagParamsBiasInstability=[ 0, 0, 0 ]  MagParamsBiasInstabilityNumerator=fractalcoef().Numerator  MagParamsBiasInstabilityDenominator=fractalcoef().Denominator  MagParamsRandomWalk=[ 0, 0, 0 ]  MagParamsNoiseType=double-sided  MagParamsTemperatureBias=[ 0, 0, 0 ]  MagParamsTemperatureScaleFactor=[ 0, 0, 0 ]
  Reshape : Reshape  OutputDimensionality=Row vector (2-D)
  Reshape2 : Reshape  OutputDimensionality=Row vector (2-D)
  Selector : Selector  InputPortWidth=3  IndexOptions=Index vector (dialog)  Indices=[3 2 1]  OutputSizes=1
  Transpose : Math  Operator=transpose
  Bus Element Out : Outport  PortName=IMU  Element=Accel
  Bus Element Out1 : Outport  PortName=IMU  Element=Gyro
  Bus Element Out2 : Outport  PortName=IMU  Element=Mag
  wires:
  Selector/1 -> Coordinate Transformation Conversion/1
  Bus Element In2/1 -> Selector/1
  IMU1/1 -> Bus Element Out/1
  IMU1/2 -> Bus Element Out1/1
  IMU1/3 -> Bus Element Out2/1
  Transpose/1 -> IMU1/3
  Gain/1 -> IMU1/1
  Coordinate Transformation Conversion/1 -> Transpose/1
  Reshape2/1 -> IMU1/2
  Bus Element In1/1 -> Reshape2/1
  Bus Element In/1 -> Reshape/1
  Reshape/1 -> Gain/1

== system Dynamics_6DOF_QUAT/Aerodynamic Model/Aero Model Enabler/If Action Subsystem1/Aerodynamic Model ==
  Thrust_mag : Inport
  V_B_rel : Inport  Port=2
  Constant : Constant  Value=Parameters.Vehicle.Cd_lumped
  D = CTV : Product
  Matrix Multiply : Product  Multiplication=Matrix(*)
  F_wind : Outport
  wires:
  Matrix Multiply/1 -> D = CTV/1
  Constant/1 -> Matrix Multiply/1
  V_B_rel/1 -> Matrix Multiply/2
  Thrust_mag/1 -> D = CTV/2
  D = CTV/1 -> F_wind/1

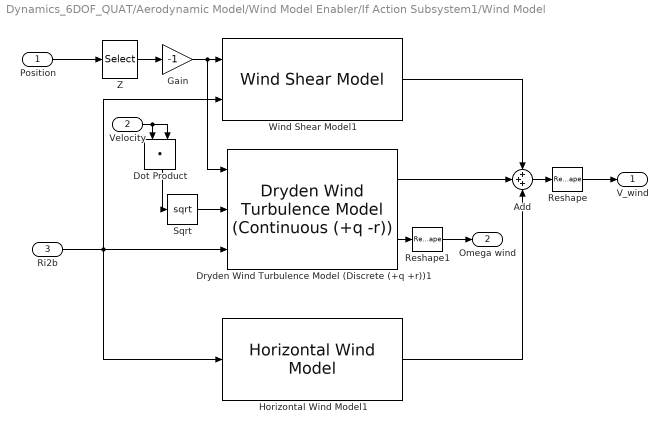
== system Dynamics_6DOF_QUAT/Aerodynamic Model/Wind Model Enabler/If Action Subsystem1/Wind Model ==
  Position : Inport
  Velocity : Inport  Port=2
  Ri2b : Inport  Port=3
  Add : Sum  Inputs=+++
  Dot Product : DotProduct  OutDataTypeStr=Inherit: Inherit via internal rule
  Dryden Wind Turbulence Model (Discrete (+q +r))1 : aerolibwind2/Dryden Wind Turbulence Model  (Continuous (+q -r))  units=Metric (MKS)  spec=MIL-F-8785C  model=Discrete Dryden (+q +r)  W20=Parameters.Simulink.wind_speed  Wdeg=Parameters.Simulink.wind_dir_deg  TurbProb=10^-2 - Light  L_high=Parameters.Simulink.wind_scale_length  Wingspan=Parameters.Simulink.wind_ref_wing_span  ts=Parameters.Simulink.wind_noise  Seed=Parameters.Simulink.wind_noise_seeds  T_on=on
  Gain : Gain  Gain=-1
  Horizontal Wind Model1 : aerolibwind2/Horizontal Wind Model  units=Metric (MKS)  Vw_source=Internal  Vwind=Parameters.Simulink.wind_speed_alt  W_source=Internal  Wdeg=Parameters.Simulink.wind_dir_alt_deg
  Reshape : Reshape  OutputDimensionality=Column vector (2-D)
  Reshape1 : Reshape  OutputDimensionality=Column vector (2-D)
  Sqrt : Sqrt
  Wind Shear Model1 : aerolibwind2/Wind Shear Model  units=Metric (MKS)  phase=Category C - Terminal Flight Phase  W_20=Parameters.Simulink.wind_speed  Wdeg=Parameters.Simulink.wind_dir_deg
  Z : Selector  InputPortWidth=3  IndexOptions=Index vector (dialog)  Indices=[3]  OutputSizes=1
  V_wind : Outport
  Omega wind : Outport  Port=2
  wires:
  Wind Shear Model1/1 -> Add/1
  Sqrt/1 -> Dryden Wind Turbulence Model (Discrete (+q +r))1/2
  Dot Product/1 -> Sqrt/1
  Gain/1 -> Wind Shear Model1/1, Dryden Wind Turbulence Model (Discrete (+q +r))1/1
  Z/1 -> Gain/1
  Horizontal Wind Model1/1 -> Add/3
  Dryden Wind Turbulence Model (Discrete (+q +r))1/1 -> Add/2
  Position/1 -> Z/1
  Velocity/1 -> Dot Product/2, Dot Product/1
  Reshape/1 -> V_wind/1
  Add/1 -> Reshape/1
  Dryden Wind Turbulence Model (Discrete (+q +r))1/2 -> Reshape1/1
  Reshape1/1 -> Omega wind/1
  Ri2b/1 -> Horizontal Wind Model1/1, Wind Shear Model1/2, Dryden Wind Turbulence Model (Discrete (+q +r))1/3

== matlab function Dynamics_6DOF_QUAT/Combine Forces and Moments/MATLAB Function1 ==
  data: v_b input; q input; omega input; tau_gyro input; T input; Tau input; g input; D input; A input; B input; k_h input; F_b output; F_e output; M_b output; m input
function [F_b, F_e, M_b] ...
    = forces_and_moments(...
    v_b, q, omega, tau_gyro,...
    T, Tau,...
    g, D, A, B, k_h,...
    m)

[F_b, F_e, M_b] ...
    = forces_and_moments(...
    v_b, q, omega, tau_gyro,...
    T, Tau,...
    g, D, A, B, k_h,...
    m);
end
